simulink model "battery_thermal_model"  (R2025a)
settings: Solver=VariableStepAuto  StartTime=0.0  StopTime=500  RelTol=1e-3
settings Model: Creator=piyus  LastModifiedBy=piyus

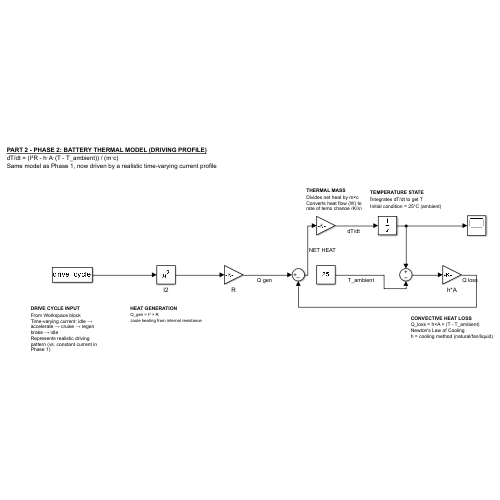
[thumbnail: Simulink's stored preview of the top-level diagram]
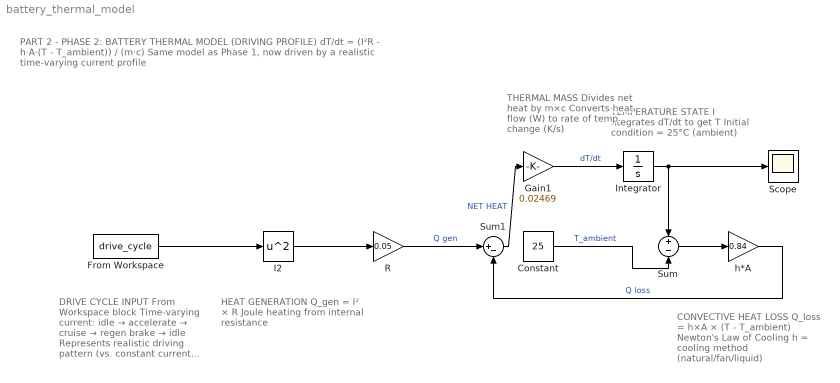
== system battery_thermal_model ==
  note: DRIVE CYCLE INPUT
      | From Workspace block
      | Time-varying current: idle → accelerate → cruise → regen brake → idle
      | Represents realistic driving pattern (vs. constant current in Phase 1)
  note: PART 2 - PHASE 2: BATTERY THERMAL MODEL (DRIVING PROFILE)
      | dT/dt = (I²R - h·A·(T - T_ambient)) / (m·c)
      | Same model as Phase 1, now driven by a realistic time-varying current profile
  note: TEMPERATURE STATE
      | I ntegrates dT/dt to get T
      | Initial condition = 25°C (ambient)
  note: THERMAL MASS
      | Divides net heat by m×c
      | Converts heat flow (W) to rate of temp change (K/s)
  note: CONVECTIVE HEAT LOSS
      | Q_loss = h×A × (T - T_ambient)
      | Newton's Law of Cooling
      | h = cooling method (natural/fan/liquid)
  note: HEAT GENERATION
      | Q_gen = I² × R
      | Joule heating from internal resistance
  Constant : Constant  Value=25
  From Workspace : FromWorkspace  VariableName=drive_cycle
  Gain1 : Gain  Gain=0.02469
  I2 : Math  Operator=square
  Integrator : Integrator  InitialCondition=25
  R : Gain  Gain=0.05
  Scope : Scope
      settings: ActiveDisplayYMinimum=24.25597571846086  ActiveDisplayYMaximum=31.696218533852253
  Sum : Sum  Inputs=+-
  Sum1 : Sum  Inputs=|+-
  h*A : Gain  Gain=0.84
  wires:
  I2/1 -> R/1
  R/1 -> Sum1/1  "Q gen"
  Constant/1 -> Sum/2  "T_ambient"
  Sum/1 -> h*A/1
  h*A/1 -> Sum1/2  "Q loss"
  Sum1/1 -> Gain1/1  "NET HEAT"
  Gain1/1 -> Integrator/1  "dT/dt"
  Integrator/1 -> Sum/1, Scope/1
  From Workspace/1 -> I2/1
